simulink model "rotating_pendulum"  (R2024a)
settings: Solver=ode45  StartTime=0.0  StopTime=20  MaxStep=0.01  RelTol=1e-8  AbsTol=1e-10
model workspace (MAT data in the model file):
  p.a = 0.3
  p.b = 0.5
  p.c = 0.1
  p.r = 0.2
  p.h = 0.15
  p.l = 0.35
  p.m = 0.25
  p.g = 9.80665
  p.alphaProfile.initialAngle = 0
  p.alphaProfile.meanRate = 1
  p.alphaProfile.amplitude = 0.2
  p.alphaProfile.frequency = 0.8
  p.alphaProfile.phase = 0
  p.betaProfile.initialAngle = 0
  p.betaProfile.meanRate = 1.6
  p.betaProfile.amplitude = 0.16
  p.betaProfile.frequency = 0.55
  p.betaProfile.phase = 0.785398163397
  p.motionFunction = []
  p.psi0 = 0.174532925199
  p.psiRate0 = 0
  p.damping = 0
  p.appliedTorque : function handle (value not decoded)
values from neighbouring files (symbols this model uses):
  p = rotpend.defaultParameters()    [build_simulink_model.m]    (also in validate_simulink_fixed_step.m; validate_simulink_model.m)
settings Model: Creator=E  LastModifiedBy=E
settings DataIOCC: SignalLogging=off

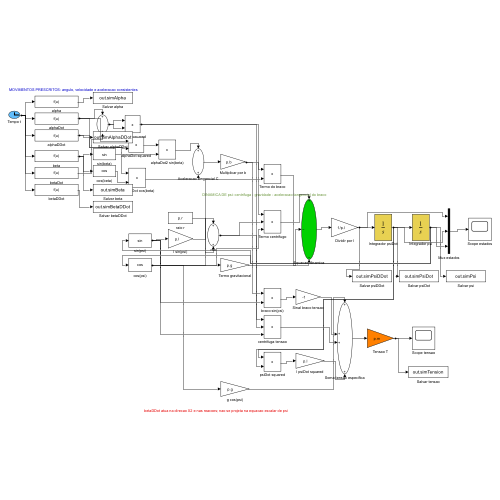
[thumbnail: Simulink's stored preview of the top-level diagram]
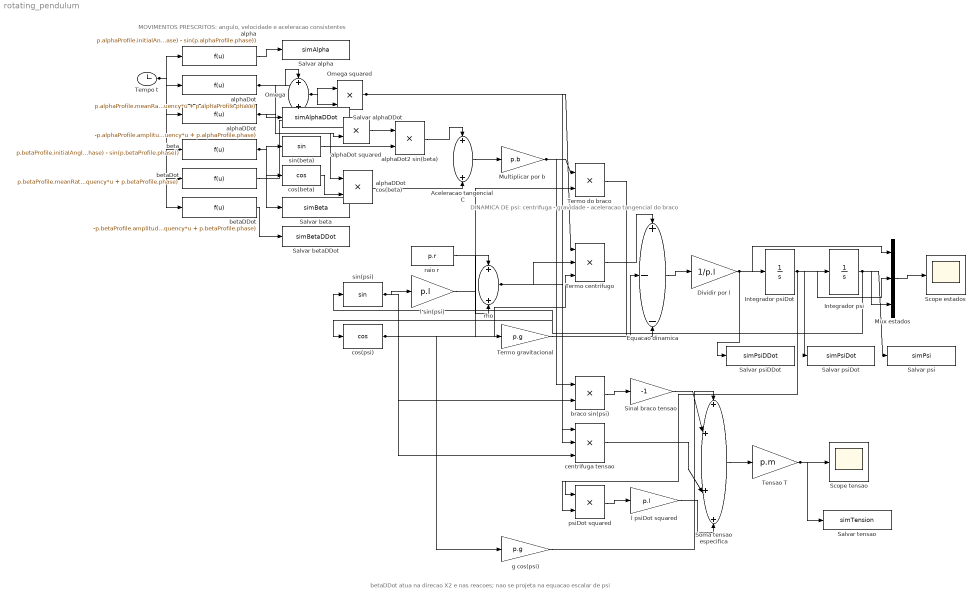
== system rotating_pendulum ==
  note: MOVIMENTOS PRESCRITOS: angulo, velocidade e aceleracao consistentes
  note: DINAMICA DE psi: centrifuga - gravidade - aceleracao tangencial do braco
  note: betaDDot atua na direcao X2 e nas reacoes; nao se projeta na equacao escalar de psi
  Aceleracao tangencial C : Sum
  Dividir por l : Gain  Gain=1/p.l
  Equacao dinamica : Sum  Inputs=+--
  Integrador psi : Integrator  InitialCondition=p.psi0
  Integrador psiDot : Integrator  InitialCondition=p.psiRate0
  Multiplicar por b : Gain  Gain=p.b
  Mux estados : Mux  Inputs=3
  Omega : Sum
  Omega squared : Product  Inputs=**
  Salvar alpha : ToWorkspace  VariableName=simAlpha  SaveFormat=Timeseries  SampleTime=-1
  Salvar alphaDDot : ToWorkspace  VariableName=simAlphaDDot  SaveFormat=Timeseries  SampleTime=-1
  Salvar beta : ToWorkspace  VariableName=simBeta  SaveFormat=Timeseries  SampleTime=-1
  Salvar betaDDot : ToWorkspace  VariableName=simBetaDDot  SaveFormat=Timeseries  SampleTime=-1
  Salvar psi : ToWorkspace  VariableName=simPsi  SaveFormat=Timeseries  SampleTime=-1
  Salvar psiDDot : ToWorkspace  VariableName=simPsiDDot  SaveFormat=Timeseries  SampleTime=-1
  Salvar psiDot : ToWorkspace  VariableName=simPsiDot  SaveFormat=Timeseries  SampleTime=-1
  Salvar tensao : ToWorkspace  VariableName=simTension  SaveFormat=Timeseries  SampleTime=-1
  Scope estados : Scope
  Scope tensao : Scope
  Sinal braco tensao : Gain  Gain=-1
  Soma tensao especifica : Sum  Inputs=++++
  Tempo t : Clock
  Tensao T : Gain  Gain=p.m
  Termo centrifugo : Product  Inputs=***
  Termo do braco : Product  Inputs=**
  Termo gravitacional : Gain  Gain=p.g
  alpha : Fcn  Expr=p.alphaProfile.initialAngle + p.alphaProfile.meanRate*u + p.alphaProfile.amplitude*(sin(p.alphaProfile.frequency*u + p.alphaProfile.phase) - sin(p.alphaProfile.phase))
  alphaDDot : Fcn  Expr=-p.alphaProfile.amplitude*p.alphaProfile.frequency^2*sin(p.alphaProfile.frequency*u + p.alphaProfile.phase)
  alphaDDot cos(beta) : Product  Inputs=**
  alphaDot : Fcn  Expr=p.alphaProfile.meanRate + p.alphaProfile.amplitude*p.alphaProfile.frequency*cos(p.alphaProfile.frequency*u + p.alphaProfile.phase)
  alphaDot squared : Product  Inputs=**
  alphaDot2 sin(beta) : Product  Inputs=**
  beta : Fcn  Expr=p.betaProfile.initialAngle + p.betaProfile.meanRate*u + p.betaProfile.amplitude*(sin(p.betaProfile.frequency*u + p.betaProfile.phase) - sin(p.betaProfile.phase))
  betaDDot : Fcn  Expr=-p.betaProfile.amplitude*p.betaProfile.frequency^2*sin(p.betaProfile.frequency*u + p.betaProfile.phase)
  betaDot : Fcn  Expr=p.betaProfile.meanRate + p.betaProfile.amplitude*p.betaProfile.frequency*cos(p.betaProfile.frequency*u + p.betaProfile.phase)
  braco sin(psi) : Product  Inputs=**
  centrifuga tensao : Product  Inputs=***
  cos(beta) : Trigonometry  Operator=cos
  cos(psi) : Trigonometry  Operator=cos
  g cos(psi) : Gain  Gain=p.g
  l psiDot squared : Gain  Gain=p.l
  l sin(psi) : Gain  Gain=p.l
  psiDot squared : Product  Inputs=**
  raio r : Constant  Value=p.r
  rho : Sum
  sin(beta) : Trigonometry
  sin(psi) : Trigonometry
  wires:
  Tempo t/1 -> alpha/1, alphaDot/1, alphaDDot/1, beta/1, betaDot/1, betaDDot/1
  beta/1 -> sin(beta)/1, cos(beta)/1, Salvar beta/1
  alphaDot/1 -> Omega/1, alphaDot squared/1, alphaDot squared/2
  betaDot/1 -> Omega/2
  Omega/1 -> Omega squared/1, Omega squared/2
  alphaDot squared/1 -> alphaDot2 sin(beta)/1
  sin(beta)/1 -> alphaDot2 sin(beta)/2
  alphaDDot/1 -> alphaDDot cos(beta)/1, Salvar alphaDDot/1
  cos(beta)/1 -> alphaDDot cos(beta)/2
  alphaDot2 sin(beta)/1 -> Aceleracao tangencial C/1
  alphaDDot cos(beta)/1 -> Aceleracao tangencial C/2
  Aceleracao tangencial C/1 -> Multiplicar por b/1
  Integrador psi/1 -> sin(psi)/1, cos(psi)/1, Mux estados/3, Salvar psi/1
  sin(psi)/1 -> l sin(psi)/1, Termo gravitacional/1, braco sin(psi)/2, centrifuga tensao/3
  l sin(psi)/1 -> rho/1
  raio r/1 -> rho/2
  Omega squared/1 -> Termo centrifugo/1, centrifuga tensao/1
  rho/1 -> Termo centrifugo/2, centrifuga tensao/2
  cos(psi)/1 -> Termo centrifugo/3, Termo do braco/2, g cos(psi)/1
  Multiplicar por b/1 -> Termo do braco/1, braco sin(psi)/1
  Termo centrifugo/1 -> Equacao dinamica/1
  Termo gravitacional/1 -> Equacao dinamica/2
  Termo do braco/1 -> Equacao dinamica/3
  Equacao dinamica/1 -> Dividir por l/1
  Dividir por l/1 -> Integrador psiDot/1, Mux estados/1, Salvar psiDDot/1
  Integrador psiDot/1 -> Integrador psi/1, psiDot squared/1, psiDot squared/2, Mux estados/2, Salvar psiDot/1
  braco sin(psi)/1 -> Sinal braco tensao/1
  psiDot squared/1 -> l psiDot squared/1
  g cos(psi)/1 -> Soma tensao especifica/1
  Sinal braco tensao/1 -> Soma tensao especifica/2
  centrifuga tensao/1 -> Soma tensao especifica/3
  l psiDot squared/1 -> Soma tensao especifica/4
  Soma tensao especifica/1 -> Tensao T/1
  Mux estados/1 -> Scope estados/1
  Tensao T/1 -> Scope tensao/1, Salvar tensao/1
  alpha/1 -> Salvar alpha/1
  betaDDot/1 -> Salvar betaDDot/1
